simulink model "playSimulink"  (R2024b)
settings: Solver=ode4  StartTime=0.0  StopTime=config.endTime  FixedStep=0.01  RelTol=1e-3
settings Model: Creator=mirkomizzoni  LastModifiedBy=mirkomizzoni

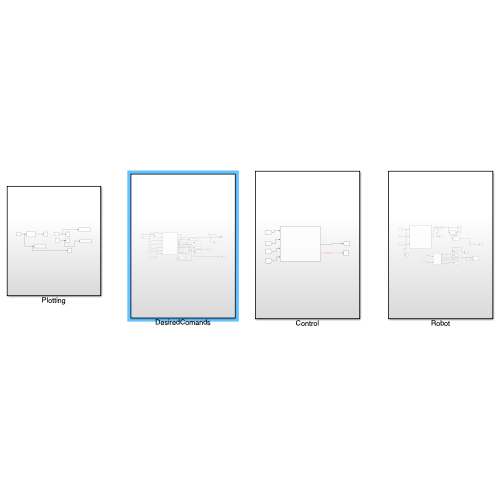
[thumbnail: Simulink's stored preview of the top-level diagram]
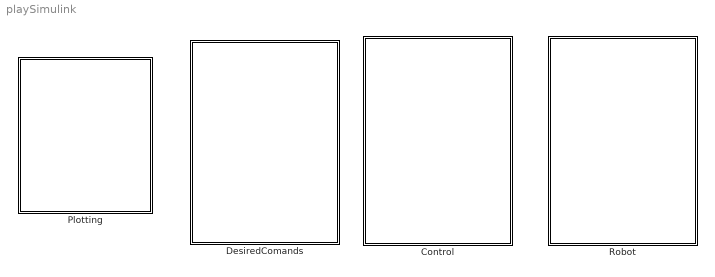
== system playSimulink ==
  Control : Subsystem
  DesiredComands : Subsystem
  Plotting : Subsystem
  Robot : Subsystem

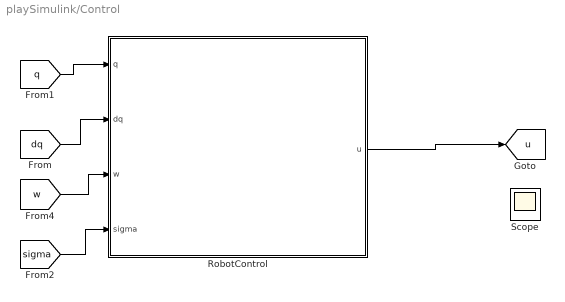
== system playSimulink/Control ==
  RobotControl : MATLAB Function  TreatAsAtomicUnit=on
  Scope : Scope
  tag scope: u=global
  wires:
  RobotControl/1(u) -> [u]
  [dq] -> RobotControl/2(dq)
  [q] -> RobotControl/1(q)
  [w] -> RobotControl/3(w)
  [sigma] -> RobotControl/4(sigma)
  ? -> Scope/1

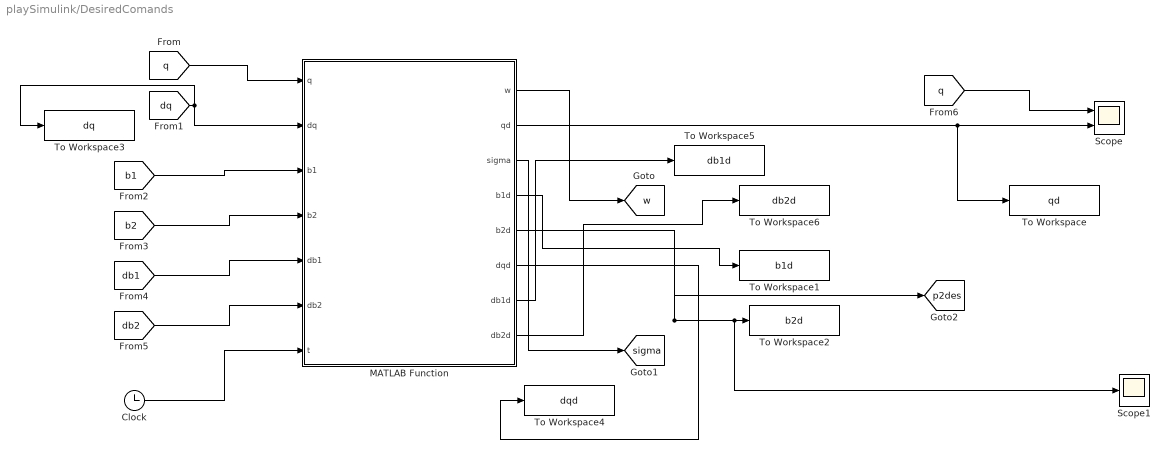
== system playSimulink/DesiredComands ==
  Clock : Clock
  MATLAB Function : MATLAB Function  TreatAsAtomicUnit=on
  Scope : Scope  NumInputPorts=2
  Scope1 : Scope
  To Workspace : ToWorkspace  VariableName=qd  SampleTime=-1
  To Workspace1 : ToWorkspace  VariableName=b1d  SampleTime=-1
  To Workspace2 : ToWorkspace  VariableName=b2d  SampleTime=-1
  To Workspace3 : ToWorkspace  VariableName=dq  SampleTime=-1
  To Workspace4 : ToWorkspace  VariableName=dqd  SampleTime=-1
  To Workspace5 : ToWorkspace  VariableName=db1d  SampleTime=-1
  To Workspace6 : ToWorkspace  VariableName=db2d  SampleTime=-1
  tag scope: p2des=global, sigma=global, w=global
  wires:
  [b1] -> MATLAB Function/3(b1)
  [db2] -> MATLAB Function/6(db2)
  [dq] -> To Workspace3/1, MATLAB Function/2(dq)
  [db1] -> MATLAB Function/5(db1)
  [b2] -> MATLAB Function/4(b2)
  MATLAB Function/1(w) -> [w]
  [q] -> MATLAB Function/1(q)
  MATLAB Function/2(qd) -> To Workspace/1, Scope/2
  MATLAB Function/3(sigma) -> [sigma]
  [q] -> Scope/1
  MATLAB Function/4(b1d) -> To Workspace1/1
  MATLAB Function/5(b2d) -> [p2des], Scope1/1, To Workspace2/1
  Clock/1 -> MATLAB Function/7(t)
  MATLAB Function/6(dqd) -> To Workspace4/1
  MATLAB Function/7(db1d) -> To Workspace5/1
  MATLAB Function/8(db2d) -> To Workspace6/1

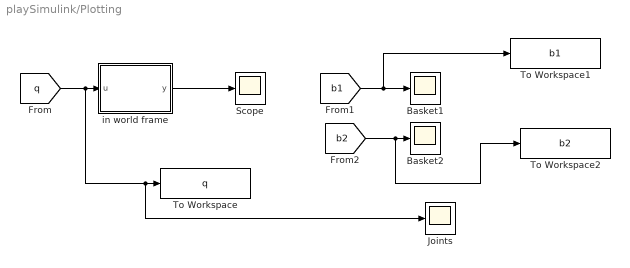
== system playSimulink/Plotting ==
  Basket1 : Scope
  Basket2 : Scope
  Joints : Scope
  Scope : Scope
  To Workspace : ToWorkspace  VariableName=q  SampleTime=-1
  To Workspace1 : ToWorkspace  VariableName=b1  SampleTime=-1
  To Workspace2 : ToWorkspace  VariableName=b2  SampleTime=-1
  in world frame : MATLAB Function  TreatAsAtomicUnit=on
  wires:
  [q] -> Joints/1, To Workspace/1, in world frame/1(u)
  in world frame/1(y) -> Scope/1
  [b1] -> To Workspace1/1, Basket1/1
  [b2] -> To Workspace2/1, Basket2/1

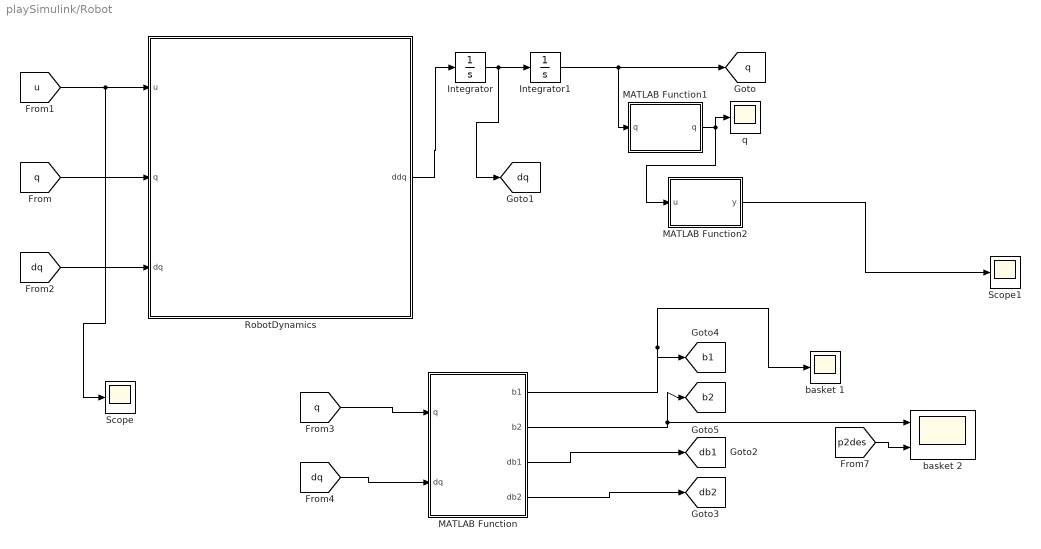
== system playSimulink/Robot ==
  Integrator : Integrator  InitialCondition=[0.1;0.1;0.1]
  Integrator1 : Integrator  InitialCondition=[0;pi/4;0]
  MATLAB Function : MATLAB Function  TreatAsAtomicUnit=on
  MATLAB Function1 : MATLAB Function  TreatAsAtomicUnit=on
  MATLAB Function2 : MATLAB Function  TreatAsAtomicUnit=on
  RobotDynamics : MATLAB Function  TreatAsAtomicUnit=on
  Scope : Scope
  Scope1 : Scope
  basket 1 : Scope
  basket 2 : Scope  NumInputPorts=2
  q : Scope
  tag scope: b1=global, b2=global, db1=global, db2=global, dq=global, q=global
  wires:
  [dq] -> RobotDynamics/3(dq)
  RobotDynamics/1(ddq) -> Integrator/1
  [u] -> Scope/1, RobotDynamics/1(u)
  Integrator/1 -> [dq], Integrator1/1
  Integrator1/1 -> MATLAB Function1/1("q "), [q]
  [q] -> RobotDynamics/2(q)
  MATLAB Function/3(db1) -> [db1]
  MATLAB Function/4(db2) -> [db2]
  MATLAB Function/1(b1) -> basket 1/1, [b1]
  MATLAB Function/2(b2) -> [b2], basket 2/1
  [q] -> MATLAB Function/1(q)
  [dq] -> MATLAB Function/2(dq)
  [p2des] -> basket 2/2
  MATLAB Function1/1(q) -> MATLAB Function2/1(u), q/1
  MATLAB Function2/1(y) -> Scope1/1

== matlab function playSimulink/Control/RobotControl ==
  data: u output; q input; dq input; w input; sigma input; config parameter
function u = fcn(q,dq,w,sigma,config)

    u = zeros(3,1);
    m1 = config.m1;
    m2 = config.m2;
    m3 = config.m3;
    l1 = config.l1;
    l2 = config.l2;
    l3 = config.l3;
    I1 = config.I1;
    I2 = config.I2;
    I3 = config.I3;
    q1 = q(1); q2 = q(2); q3= q(3);
    dq1 = dq(1); dq2 = dq(2); dq3= dq(3);
    b = drift_s(I1,I2,I3,dq1,dq2,dq3,l1,l2,l3,m1,m2,m3,q1,q2,q3);
    
    Bmat = allocMatrixInt_s(I1,I2,I3,l1,l2,l3,m1,m2,m3,q1,q2,q3);
    %sigma = [1 1 1 0 0 0 0];
    S = diag(sigma);
    activeIdx = find(sigma);
    Gamma = S(activeIdx,:);
    %A = Gamma * Bmat;
    sigma
    %u = A^-1*(-Gamma*b+Gamma*w);
   
    if ~isempty(activeIdx)
            Gamma = S(activeIdx,:);
            A = Gamma * Bmat;
            rhs = -Gamma*b + Gamma*w;
        
            if size(A,1) == size(A,2)
               u = A \ rhs;
            end
           
    end
       
    % legend
  
end

== matlab function playSimulink/Robot/RobotDynamics ==
  data: u input; ddq output size=[3,1]; q input; dq input; config parameter
function ddq = fcn(u,q,dq,config)

    m1 = config.m1;
    m2 = config.m2;
    m3 = config.m3;
    l1 = config.l1;
    l2 = config.l2;
    l3 = config.l3;
    I1 = config.I1;
    I2 = config.I2;
    I3 = config.I3;

    u1 = u(1); u2 = u(2); u3= u(3);
    q1 = q(1); q2 = q(2); q3= q(3);
    dq1 = dq(1); dq2 = dq(2); dq3= dq(3);
    ddq = ddq_s(I1,I2,I3,dq1,dq2,dq3,l1,l2,l3,m1,m2,m3,q2,q3,u1,u2,u3);


end

== matlab function playSimulink/DesiredComands/MATLAB Function ==
  data: q input; w output; dq input; b1 input; b2 input; db1 input size=[2,1]; db2 input size=[2,1]; qd output; sigma output; b1d output; b2d output; t input; config parameter; dqd output; db1d output; db2d output
function [w, qd, sigma, b1d, b2d, dqd, db1d, db2d] = desCmd(q, dq, b1, b2, db1, db2, t, config)

    %% ================== DEFAULT REFERENCES ==================
    qd   = [0; pi/8; pi/4];
    dqd  = [0; 0; 0];
    ddqd = [0; 0; 0];

    b1d  = [0; 0];
    b2d  = [4.3; 3.5];

    db1d = [0; 0];
    db2d = [0; 0];

    switching_instants = config.switching_instants;
    p_des = config.p_des;

    ydot = [dq; db1; db2];

    y_d_ddot = [ddqd; 0; 0; 0; 0];
    y_d_dot  = [dqd; db1d; db2d];

    %% ================== DEFAULT SIGMA ==================
    idx = 2;
    sigma = zeros(1,7);
    sigma(3) = 1;
    sigma(idx+4) = 1;
    sigma(idx+5) = 1;

    %% ================== INTERVAL 1 ==================
    if t <= switching_instants(2)

        [~, idx] = selectClosestBasket(p_des(:,1), b1, b2);

        sigma = zeros(1,7);
        sigma(3) = 1;

        if idx == 1
            b1d = p_des(:,1);
            db1d = [0; 0];

            sigma(4) = 1;
            sigma(5) = 1;
        else
            b2d = p_des(:,1);
            db2d = [0; 0];

            sigma(6) = 1;
            sigma(7) = 1;
        end

        disp('Time interval 1: Closest basket');
        disp(idx);
    end

    %% ================== INTERVAL 2: MOVING ITEM ON BOUNDED CIRCLE ==================
    if t >= switching_instants(2) && t <= switching_instants(3)

        [~, idx] = selectClosestBasket(p_des(:,2), b1, b2);

        sigma = zeros(1,7);
        sigma(2) = 1;

        t0 = switching_instants(2);
        tf = switching_instants(3);
        T  = tf - t0;

        % Bounded circular trajectory.
        %
        % This shifted-circle parametrization starts exactly at p_des(:,2):
        %
        %   p_item(t0) = pc.
        %
        % It also returns to pc at the end of the interval if one full
        % revolution is completed.
        pc = p_des(:,2);
        r  = 0.25;
        omega = 2*pi/T;

        theta = omega*(t - t0);

        p_item = pc + r*[cos(theta) - 1; sin(theta)];
        v_item = r*omega*[-sin(theta); cos(theta)];

        if idx == 1
            b1d = p_item;
            db1d = v_item;

            sigma(4) = 1;
            sigma(5) = 1;
        else
            b2d = p_item;
            db2d = v_item;

            sigma(6) = 1;
            sigma(7) = 1;
        end

        y_d_dot = [dqd; db1d; db2d];

        disp('Time interval 2: Moving circular item, closest basket');
        disp(idx);
    end

    %% ================== INTERVAL 3: MOVING ITEM ON BOUNDED CIRCLE ==================
    if t >= switching_instants(3) && t <= switching_instants(4)

        sigma = zeros(1,7);
        sigma(3) = 1;
        sigma(4) = 1;
        sigma(5) = 1;

        t0 = switching_instants(3);
        tf = switching_instants(4);
        T  = tf - t0;

        % Bounded shifted-circle trajectory starting exactly at p_des(:,3).
        pc = p_des(:,3);
        r  = 0.25;
        omega = 2*pi/T;

        theta = omega*(t - t0);

        p_item = pc + r*[cos(theta) - 1; sin(theta)];
        v_item = r*omega*[-sin(theta); cos(theta)];

        b1d = p_item;
        db1d = v_item;

        y_d_dot = [dqd; db1d; db2d];

        disp('Time interval 3: Moving circular item with gripper 1');
    end

    %% ================== INTERVAL 4 ==================
    if t >= switching_instants(4) && t <= switching_instants(5)

        [~, idx] = selectClosestBasket(p_des(:,4), b1, b2);

        sigma = zeros(1,7);
        sigma(3) = 1;

        if idx == 1
            b1d = p_des(:,4);
            db1d = [0; 0];

            sigma(4) = 1;
            sigma(5) = 1;
        else
            b2d = p_des(:,4);
            db2d = [0; 0];

            sigma(6) = 1;
            sigma(7) = 1;
        end

        disp('Time interval 4: Closest basket');
        disp(idx);
    end

    %% ================== INTERVAL 5 ==================
    if t >= switching_instants(5) && t <= switching_instants(6)

        [~, idx] = selectClosestBasket(p_des(:,5), b1, b2);

        sigma = zeros(1,7);
        sigma(1) = 1;

        if idx == 1
            b1d = p_des(:,5);
            db1d = [0; 0];

            sigma(4) = 1;
            sigma(5) = 1;
        else
            b2d = p_des(:,5);
            db2d = [0; 0];

            sigma(6) = 1;
            sigma(7) = 1;
        end

        disp('Time interval 5: Closest basket');
        disp(idx);
    end

    %% ================== INTERVAL 6: RETURN CONFIGURATION ==================
    if t >= switching_instants(6)

        sigma = [1 1 1 0 0 0 0];

        qd = [0; pi/4; 0];
        dqd = [0; 0; 0];

        b1d = [0; 0];
        b2d = [4.3; 3.5];

        db1d = [0; 0];
        db2d = [0; 0];

        y_d_dot = [dqd; db1d; db2d];

        disp('Time interval 6: End of the task');
    end

    %% ================== CONTROL LAW ==================
    angle_error = atan2(sin(qd - q), cos(qd - q));

    pos_error = [
        angle_error;
        b1d - b1;
        b2d - b2
    ];

    % Update desired first derivative after all interval logic.
    y_d_dot = [dqd; db1d; db2d];

    k1 = config.k2;
    k0 = config.k1;

    w = y_d_ddot + k1*(y_d_dot - ydot) + k0*pos_error;

end

function [b_closest, idx] = selectClosestBasket(p_des, b1, b2)
    % SELECTCLOSESTBASKET returns index 1 or 2 and the closest basket position.
    p_des = p_des(:);
    b1 = b1(:);
    b2 = b2(:);

    d1 = sum((p_des - b1).^2);
    d2 = sum((p_des - b2).^2);

    if d1 <= d2
        b_closest = b1;
        idx = int8(1);
    else
        b_closest = b2;
        idx = int8(2);
    end
end

== matlab function playSimulink/Robot/MATLAB Function ==
  data: q input; dq input; b1 output; b2 output; db1 output; db2 output; config parameter
function [b1,b2,db1,db2]= fcn(q,dq,config)
    

    l1 = config.l1;
    l2 = config.l2;
    l3 = config.l3;
    dq1 = dq(1); dq2 = dq(2); dq3= dq(3);
    q1 = q(1); q2 = q(2); q3= q(3);

    b1 = [l1*cos(q1) + l2/2*cos(q1+q2) ;
      l1*sin(q1)+ l2/2*sin(q1+q2)];

    b2 = [l1*cos(q1) + l2*cos(q1+q2) + l3*cos(q1+q2+q3);
          l1*sin(q1) + l2*sin(q1+q2) + l3*sin(q1+q2+q3)];
    db1 = pb1dot_s(dq1,dq2,l1,l2,q1,q2);
    db2 = pb2dot_s(dq1,dq2,dq3,l1,l2,l3,q1,q2,q3);


end

== matlab function playSimulink/Robot/MATLAB Function1 ==
  data: q input; q output
function q = fcn(q)
    q = atan2(sin( q), cos(q));  % 3x1
end

== matlab function playSimulink/Plotting/in world frame ==
  data: u input; y output
function y = fcn(u)

y = [rad2deg(u(1));rad2deg(u(1)+u(2));rad2deg(u(1)+u(2)+u(3))];

== matlab function playSimulink/Robot/MATLAB Function2 ==
  data: u input; y output
function y = fcn(u)

y = norm(u);

end
